simulink model "distributed_project_block_prev"  (R2022b)
settings: Solver=VariableStepAuto  StartTime=0.0  StopTime=10.0  RelTol=1e-3
values from neighbouring files (symbols this model uses):
  A_bar = kron(eye(N), A)    [distributed_project.m]
  B_bar = kron(eye(N), B)    [distributed_project.m]
  C_bar = kron(eye(N), C)    [distributed_project.m]
  D_bar = kron(eye(N), D)    [distributed_project.m]
  Gamma_cap_bar = kron(eye(N), gamma_cap)    [distributed_project.m]
  h_bar = [2;4;2;4;2;4;2;4;]    [distributed_project.m]
  K_bar = kron(eye(N), K)    [distributed_project.m]
  L_bar = kron(L,eye(n))    [distributed_project.m]
  M1 = [1 0 0 0 0 0 0 0 ... (first row only)    [distributed_project.m]
  M2 = [0 0 0 0 0 0 0 0 ... (first row only)    [distributed_project.m]
  M3 = [0 0 0 0 0 0 0 0 ... (first row only)    [distributed_project.m]
  M4 = [0 0 0 0 0 0 0 0 ... (first row only)    [distributed_project.m]
  P_bar = kron(eye(N), P)    [distributed_project.m]
libraries: matrix_library x4
settings Model: Creator=BALA SUBRAHMANYAM  LastModifiedBy=USER
settings OptimizationCC: ReuseModelBlockBuffer=on

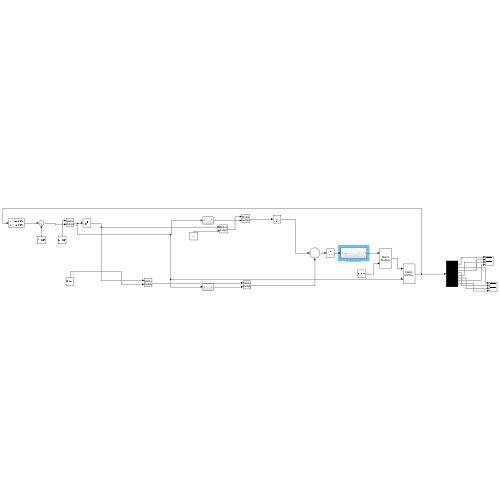
[thumbnail: Simulink's stored preview of the top-level diagram]
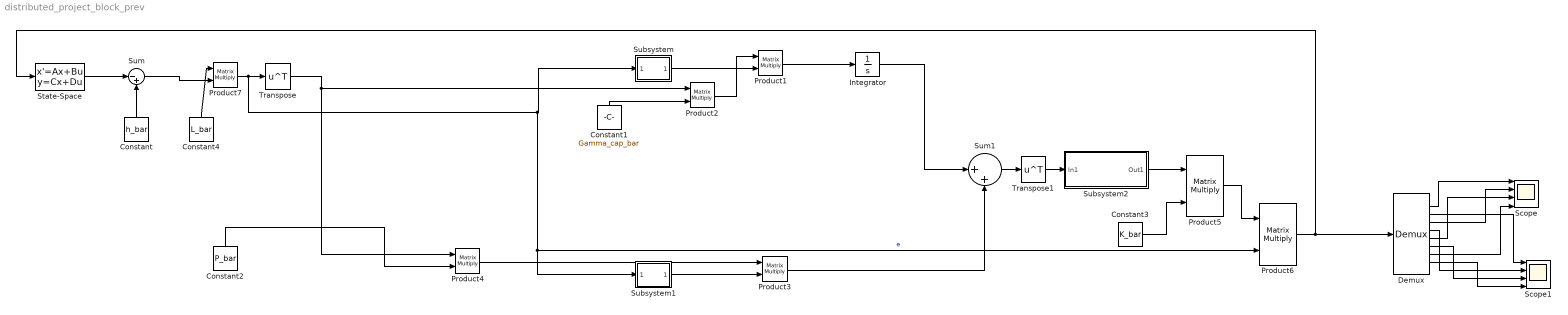
== system distributed_project_block_prev ==
  Constant : Constant  Value=h_bar
  Constant1 : Constant  Value=Gamma_cap_bar
  Constant2 : Constant  Value=P_bar
  Constant3 : Constant  Value=K_bar
  Constant4 : Constant  Value=L_bar
  Demux : Demux  Outputs=8
  Integrator : Integrator
  Product{1..7} (7 alike) : Product  Multiplication=Matrix(*)
  Scope : Scope  NumInputPorts=4
  Scope1 : Scope  NumInputPorts=4
  State-Space : StateSpace  A=A_bar  B=B_bar  C=C_bar  D=D_bar  InitialCondition=0
  Subsystem : Subsystem
  Subsystem1 : Subsystem
  Subsystem2 : Subsystem
  Sum : Sum  Inputs=|-+
  Sum1 : Sum  Inputs=|++
  Transpose : Math  Operator=transpose
  Transpose1 : Math  Operator=transpose
  wires:
  State-Space/1 -> Sum/1
  Constant/1 -> Sum/2
  Product7/1 -> Subsystem1/1(In1), Product6/2, Subsystem/1(In1), Transpose/1  "e"
  Transpose/1 -> Product4/1, Product2/1
  Product1/1 -> Integrator/1
  Product3/1 -> Sum1/2
  Constant2/1 -> Product4/2
  Constant1/1 -> Product2/2
  Product2/1 -> Product1/1
  Product4/1 -> Product3/1
  Integrator/1 -> Sum1/1
  Subsystem/1(Out1) -> Product1/2
  Subsystem1/1(Out1) -> Product3/2
  Sum1/1 -> Transpose1/1
  Transpose1/1 -> Subsystem2/1(In1)
  Subsystem2/1(Out1) -> Product5/1
  Constant3/1 -> Product5/2
  Product5/1 -> Product6/1
  Product6/1 -> Demux/1, State-Space/1
  Demux/1 -> Scope/1
  Demux/3 -> Scope/2
  Demux/5 -> Scope/3
  Demux/7 -> Scope/4
  Demux/2 -> Scope1/1
  Demux/4 -> Scope1/2
  Demux/6 -> Scope1/3
  Demux/8 -> Scope1/4
  Sum/1 -> Product7/2
  Constant4/1 -> Product7/1

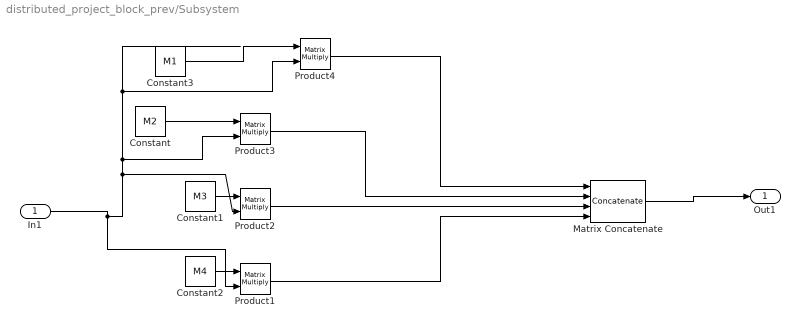
== system distributed_project_block_prev/Subsystem ==
  In1 : Inport
  Constant : Constant  Value=M2
  Constant1 : Constant  Value=M3
  Constant2 : Constant  Value=M4
  Constant3 : Constant  Value=M1
  Matrix Concatenate : Concatenate  NumInputs=4  Mode=Multidimensional array  ConcatenateDimension=2
  Product{1..4} (4 alike) : Product  Multiplication=Matrix(*)
  Out1 : Outport
  wires:
  In1/1 -> Product1/2, Product3/2, Product4/2, Product2/2
  Product4/1 -> Matrix Concatenate/1
  Product3/1 -> Matrix Concatenate/2
  Product2/1 -> Matrix Concatenate/3
  Product1/1 -> Matrix Concatenate/4
  Matrix Concatenate/1 -> Out1/1
  Constant/1 -> Product3/1
  Constant3/1 -> Product4/1
  Constant2/1 -> Product1/1
  Constant1/1 -> Product2/1

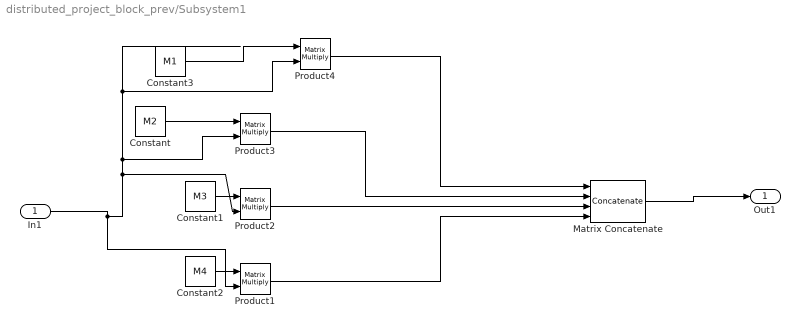
== system distributed_project_block_prev/Subsystem1 ==
  In1 : Inport
  Constant : Constant  Value=M2
  Constant1 : Constant  Value=M3
  Constant2 : Constant  Value=M4
  Constant3 : Constant  Value=M1
  Matrix Concatenate : Concatenate  NumInputs=4  Mode=Multidimensional array  ConcatenateDimension=2
  Product{1..4} (4 alike) : Product  Multiplication=Matrix(*)
  Out1 : Outport
  wires:
  In1/1 -> Product1/2, Product3/2, Product4/2, Product2/2
  Product4/1 -> Matrix Concatenate/1
  Product3/1 -> Matrix Concatenate/2
  Product2/1 -> Matrix Concatenate/3
  Product1/1 -> Matrix Concatenate/4
  Matrix Concatenate/1 -> Out1/1
  Constant/1 -> Product3/1
  Constant3/1 -> Product4/1
  Constant2/1 -> Product1/1
  Constant1/1 -> Product2/1

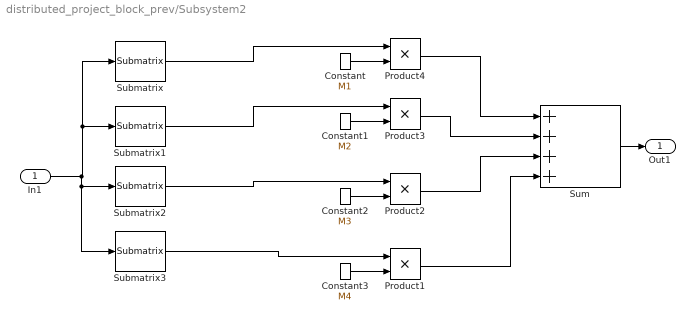
== system distributed_project_block_prev/Subsystem2 ==
  In1 : Inport
  Constant : Constant  Value=M1
  Constant1 : Constant  Value=M2
  Constant2 : Constant  Value=M3
  Constant3 : Constant  Value=M4
  Product{1..4} (4 alike) : Product
  Submatrix : matrix_library/Submatrix  RowSpan=One row  RowStartMode=First  RowStartIndex=1  RowEndMode=Last  RowEndIndex=1  ColSpan=One column  ColStartMode=First  ColStartIndex=1  ColEndMode=Last  ColEndIndex=1
  Submatrix1 : matrix_library/Submatrix  RowSpan=One row  RowStartMode=Index  RowStartIndex=2  RowEndMode=Last  RowEndIndex=1  ColSpan=One column  ColStartMode=First  ColStartIndex=1  ColEndMode=Last  ColEndIndex=1
  Submatrix2 : matrix_library/Submatrix  RowSpan=One row  RowStartMode=Index  RowStartIndex=3  RowEndMode=Last  RowEndIndex=1  ColSpan=One column  ColStartMode=First  ColStartIndex=1  ColEndMode=Last  ColEndIndex=1
  Submatrix3 : matrix_library/Submatrix  RowSpan=One row  RowStartMode=Index  RowStartIndex=4  RowEndMode=Last  RowEndIndex=1  ColSpan=One column  ColStartMode=First  ColStartIndex=1  ColEndMode=Last  ColEndIndex=1
  Sum : Sum  Inputs=++++
  Out1 : Outport
  wires:
  In1/1 -> Submatrix2/1, Submatrix3/1, Submatrix1/1, Submatrix/1
  Constant/1 -> Product4/2
  Constant1/1 -> Product3/2
  Constant2/1 -> Product2/2
  Constant3/1 -> Product1/2
  Submatrix/1 -> Product4/1
  Submatrix1/1 -> Product3/1
  Submatrix2/1 -> Product2/1
  Submatrix3/1 -> Product1/1
  Product4/1 -> Sum/1
  Product3/1 -> Sum/2
  Product2/1 -> Sum/3
  Product1/1 -> Sum/4
  Sum/1 -> Out1/1
